simulink model "phase shifted fullbridge converter"  (R2024b)
settings: Solver=ode23t  StartTime=0.0  StopTime=.1  RelTol=1e-3
values from neighbouring files (symbols this model uses):
  c = del_i*d/(del_v*fs)    (= 0.000333333333333)    [psfbc_code.m]
  fs = 100*10^3    (= 100000)    [psfbc_code.m]
  l = (vi*n-vo)*d/(fs*del_i)    (= 1.2e-06)    [psfbc_code.m]
  n1 = vi    (= 400)    [psfbc_code.m]
  n2 = vy    (= 15)    [psfbc_code.m]
  po = 600    [psfbc_code.m]
  r = vo/io    (= 0.24)    [psfbc_code.m]
  vi = 400    [psfbc_code.m]
libraries: spsDiodeLib x4, spsMosfetLib x4, spsSeriesRLCBranchLib x3, spsVoltageMeasurementLib x2, spsCurrentMeasurementLib x1, spsDCVoltageSourceLib x1, spsLinearTransformerLib x1, slpidlib x1, spspowerguiLib x1
settings Model: Creator=91798  LastModifiedBy=91798

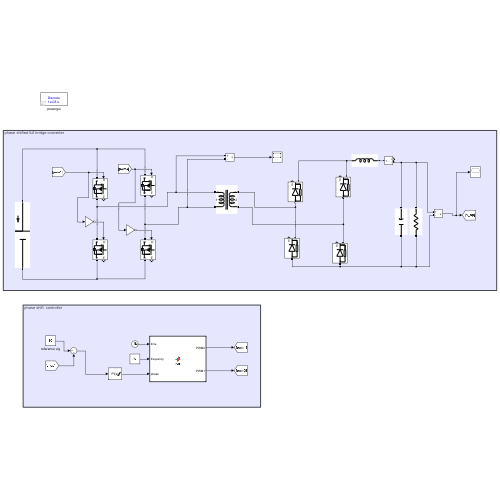
[thumbnail: Simulink's stored preview of the top-level diagram]
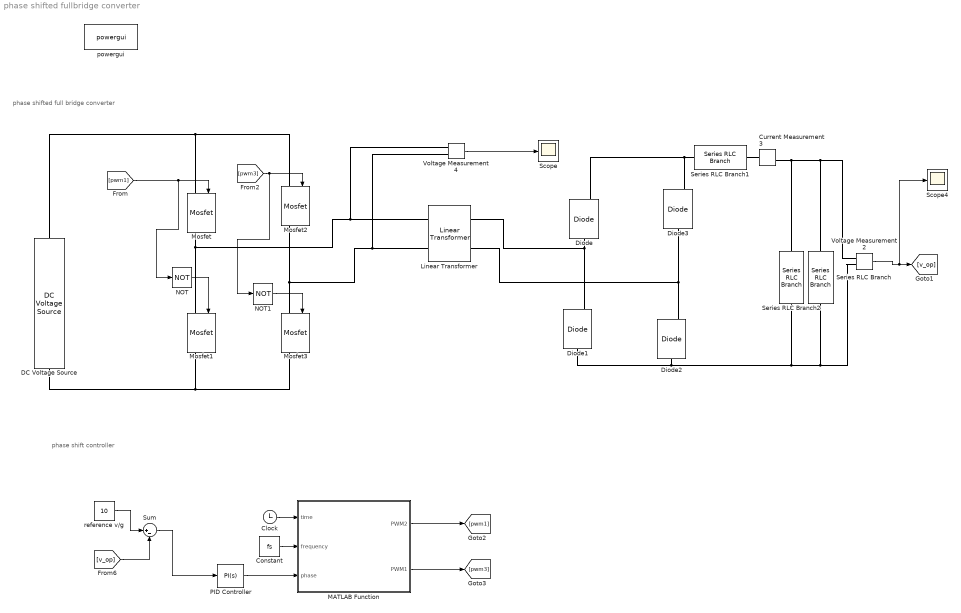
== system phase shifted fullbridge converter ==
  note: phase shifted full bridge converter
  note: phase shift controller
  Clock : Clock
  Constant : Constant  Value=fs
  Current Measurement3 : spsCurrentMeasurementLib/Current Measurement  PhasorSimulation=off  OutputType=Complex  PSBequivalent=0
  DC Voltage Source : spsDCVoltageSourceLib/DC Voltage Source  Amplitude=vi  Measurements=None
  Diode{,1..3} (4 alike) : spsDiodeLib/Diode  Ron=0.001  Lon=0  Vf=0.8  IC=0  UseSnubber=0  Rs=500  Cs=250e-9  Measurements=on
  Linear Transformer : spsLinearTransformerLib/Linear Transformer  UNITS=SI  NominalPower=[ po fs ]  winding1=[n1 1e-9 1e-10]  winding2=[n2 1e-9 1e-10]  ThreeWindings=off  winding3=[3.15e+05 0.7938 0.084225]  RmLm=[4e+06 2866]  Measurements=None  DataType=on
  MATLAB Function : MATLAB Function  TreatAsAtomicUnit=on
  Mosfet{,1..3} (4 alike) : spsMosfetLib/Mosfet  Ron=0.1  Lon=0  Rd=0.01  Vfd=0  IC=0  Rs=1e5  Cs=inf  Measurements=on
  NOT : Logic  Operator=NOT  IconShape=distinctive  AllPortsSameDT=off  OutDataTypeStr=boolean
  NOT1 : Logic  Operator=NOT  IconShape=distinctive  AllPortsSameDT=off  OutDataTypeStr=boolean
  PID Controller : slpidlib/PID Controller  Controller=PI  Form=Parallel  TimeDomain=Continuous-time  UseExternalTs=off  SampleTime=-1  IntegratorMethod=Forward Euler  FilterMethod=Forward Euler  ControllerParametersSource=internal  P=100000  I=500  UseKiTs=off  D=0  UseExternalDerivativeSource=off  N=100  UseFilter=on  TunerSelectOption=Transfer Function Based (PID Tuner App)  InitialConditionSource=internal  InitialConditionForIntegrator=0  InitialConditionForFilter=0  DifferentiatorICPrevScaledInput=0  ExternalReset=none  TrackingMode=off  Kt=1  LimitOutput=on  SatLimitsSource=internal  UpperSaturationLimit=180  LowerSaturationLimit=0  LinearizeAsGain=off  AntiWindupMode=none  Kb=1  LimitIntegrator=off  UpperIntegratorSaturationLimit=180  LowerIntegratorSaturationLimit=0  POutMin=[]  POutMax=[]  IOutMin=[]  IOutMax=[]  DOutMin=[]  DOutMax=[]  NOutMin=[]  NOutMax=[]  SumOutMin=[]  SumOutMax=[]  SaturationOutMin=[]  SaturationOutMax=[]  PParamMin=[]  PParamMax=[]  IParamMin=[]  IParamMax=[]  DParamMin=[]  DParamMax=[]  NParamMin=[]  NParamMax=[]  KbParamMin=[]  KbParamMax=[]  KtParamMin=[]  KtParamMax=[]  KbOutMin=[]  KbOutMax=[]  KtOutMin=[]  KtOutMax=[]  IntegratorOutMin=[]  IntegratorOutMax=[]  FilterOutMin=[]  FilterOutMax=[]  SumI1OutMin=[]  SumI1OutMax=[]  SumI2OutMin=[]  SumI2OutMax=[]  SumI3OutMin=[]  SumI3OutMax=[]  SumI4OutMin=[]  SumI4OutMax=[]  SumDOutMin=[]  SumDOutMax=[]  DifferentiatorOutMin=[]  DifferentiatorOutMax=[]  FilterDiffOutCoefMin=[]  FilterDiffOutCoefMax=[]  ReciprocalOutMin=[]  ReciprocalOutMax=[]  SumDenOutMin=[]  SumDenOutMax=[]  SumNumOutMin=[]  SumNumOutMax=[]  DivideOutMin=[]  DivideOutMax=[]  UdiffTsProdOutMin=[]  UdiffTsProdOutMax=[]  NTsProdOutMin=[]  NTsProdOutMax=[]  UintegralTsProdOutMin=[]  UintegralTsProdOutMax=[]  UngainTsProdOutMin=[]  UngainTsProdOutMax=[]  ClampingZeroOutDataTypeStr=Inherit: Inherit via back propagation  ClampingZeroOutMin=[]  ClampingZeroOutMax=[]  FilterDenConstantOutDataTypeStr=Inherit: Inherit via back propagation  FilterDenConstantOutMin=[]  FilterDenConstantOutMax=[]  PCopyOutDataTypeStr=Inherit: Inherit via back propagation  PCopyOutMin=[]  PCopyOutMax=[]  NCopyOutDataTypeStr=Inherit: Inherit via back propagation  NCopyOutMin=[]  NCopyOutMax=[]  IntegratorContinuousStateAttributes=''  IntegratorStateMustResolveToSignalObject=off  IntegratorRTWStateStorageClass=Auto  FilterContinuousStateAttributes=''  FilterStateMustResolveToSignalObject=off  FilterRTWStateStorageClass=Auto  ParallelPVariant=InternalParameters  IdealPVariant=Disabled  IVariant=InternalParameters  DVariant=Disabled  IntegratorVariant=Continuous  SatVariant=Enabled  AWVariant=Passthrough  PCopyVariant=Disabled  TRVariant=Disabled  FdbkBlocksVariant=Forward  IdealPFdbkVariant=Disabled  SatFdbkVariant=Disabled  DerivativeFilterVariant=Disabled  NVariant=Disabled  NCopyVariant=Disabled_SignalSpec  FilterICVariant=Disabled  IntegratorICVariant=InternalICs  ExternalResetVariant=Disabled  TRSumVariant=Passthrough  SumFdbkVariant=Disabled  SumVariant=Sum_PI  TsampFilterVariant=InternalTs  TsampNgainVariant=Passthrough  TsampIntegralVariant=Disabled_SignalSpec  ExternalSaturationOutDataTypeStr=Inherit: Same as second input  DerivativeSourceVariant=Disabled  PreIntVariant=InternalPreInt
  Scope : Scope
  Scope4 : Scope
  Series RLC Branch : spsSeriesRLCBranchLib/Series RLC Branch  LConnTagsString=__new0  RConnTagsString=__new0  BranchType=R  Resistance=r  Inductance=1e-3  SetiL0=off  InitialCurrent=0  Capacitance=1e-6  Setx0=off  InitialVoltage=0  Measurements=None
  Series RLC Branch1 : spsSeriesRLCBranchLib/Series RLC Branch  LConnTagsString=__new0  RConnTagsString=__new0  BranchType=L  Resistance=r  Inductance=l  SetiL0=off  InitialCurrent=0  Capacitance=1e-6  Setx0=off  InitialVoltage=0  Measurements=None
  Series RLC Branch2 : spsSeriesRLCBranchLib/Series RLC Branch  LConnTagsString=__new0  RConnTagsString=__new0  BranchType=C  Resistance=r  Inductance=l  SetiL0=off  InitialCurrent=0  Capacitance=c  Setx0=off  InitialVoltage=0  Measurements=None
  Sum : Sum  Inputs=|+-
  Voltage Measurement2 : spsVoltageMeasurementLib/Voltage Measurement  PhasorSimulation=off  OutputType=Complex  PSBequivalent=0
  Voltage Measurement4 : spsVoltageMeasurementLib/Voltage Measurement  PhasorSimulation=off  OutputType=Complex  PSBequivalent=0
  powergui : spspowerguiLib/powergui  Priority=1  SimulationMode=Discrete  SampleTime=1e-8  frequency=60  Iterations=50  frequencyindice=0  Pbase=100e6  ErrMax=1e-4  UnitsV=kV  UnitsW=MW  buscounter=0  FunctionMessages=off  echomessages=off  EnableUseOfTLC=off  CurrentSourceSwitches=off  DisableSnubberDevices=off  DisableRonSwitches=off  DisableVfSwitches=off  DisplayEquations=off  AutomaticDiscreteSolvers=off  SolverType=Tustin/Backward Euler (TBE)  Interpol=off  ExternalGateDelay=off  methode=off  Ts=100  x0status=blocks  SPID=on  SwTol=0  HookPort=off  NonlinearTolerance=1e-4  nMaxIteration=100  ContinueOnMaxIteration=off  RestoreLinks=warning  ResistiveCurrentMeasurement=off  Frange=[0:2:500]  Ylog=off  Xlog=on  ShowGrid=off  save=off  variable=ZData  structure=0  ZoomFFT=off  StartTime=0.0  cycles=1  DisplayStyle=1  fundamental=60  FreqAxis=off  MaxFrequency=1000  frequencyindicesteady=1  RmsSteady=1  display=off
  reference v/g : Constant  Value=10
  wires:
  [pwm1] -> Mosfet/1, NOT/1
  Voltage Measurement4/1 -> Scope/1
  NOT/1 -> Mosfet1/1
  NOT1/1 -> Mosfet3/1
  [pwm3] -> Mosfet2/1, NOT1/1
  Voltage Measurement2/1 -> Scope4/1, [v_op]
  reference v/g/1 -> Sum/1
  [v_op] -> Sum/2
  Sum/1 -> PID Controller/1
  Clock/1 -> MATLAB Function/1(time)
  Constant/1 -> MATLAB Function/2(frequency)
  PID Controller/1 -> MATLAB Function/3(phase)
  MATLAB Function/1(PWM2) -> [pwm1]
  MATLAB Function/2(PWM1) -> [pwm3]
  connections:
  Voltage Measurement2/LConn1 -- Series RLC Branch2/RConn1 -- Current Measurement3/RConn1 -- Series RLC Branch/LConn1
  Linear Transformer/RConn2 -- Diode3/LConn1 -- Diode2/RConn1
  Mosfet2/RConn1 -- Mosfet3/LConn1 -- Voltage Measurement4/LConn2 -- Linear Transformer/LConn2
  Voltage Measurement2/LConn2 -- Series RLC Branch2/LConn1 -- Diode2/LConn1 -- Diode1/LConn1 -- Series RLC Branch/RConn1
  Mosfet1/LConn1 -- Mosfet/RConn1 -- Voltage Measurement4/LConn1 -- Linear Transformer/LConn1
  DC Voltage Source/LConn1 -- Mosfet3/RConn1 -- Mosfet1/RConn1
  Diode/RConn1 -- Diode3/RConn1 -- Series RLC Branch1/LConn1
  Linear Transformer/RConn1 -- Diode1/RConn1 -- Diode/LConn1
  DC Voltage Source/RConn1 -- Mosfet2/LConn1 -- Mosfet/LConn1
  Current Measurement3/LConn1 -- Series RLC Branch1/RConn1

== matlab function phase shifted fullbridge converter/MATLAB Function ==
  data: time input; PWM2 output; frequency input; phase input; PWM1 output
function [ PWM2, PWM1] = fcn(time, frequency, phase)
    Tswitching = 1 / frequency;  % Calculate switching period
    PWM1 = 0; % Initialize PWM1 signal
    PWM2 = 0; % Initialize PWM2 signal
    
    % Generate PWM1 signal
    y1 = mod(time, Tswitching); % Calculate the current time within the switching period
    if y1 < Tswitching / 2       % Compare to half the period for a 50% duty cycle
        PWM1 = 1;               % Set PWM1 high
    end
    
    % Calculate phase shift in time
    t_phi = (Tswitching / 360)* phase ; % Convert phase (degrees) into time
    
    % Generate PWM2 signal
    y2 = mod(time + t_phi, Tswitching); % Shift time by the phase shift
    if y2 < Tswitching / 2             % Similar comparison for PWM2
        PWM2 = 1;                      % Set PWM2 high
    end
end
